simulink model "inverter_hil"  (R2024b)
settings: Solver=FixedStepDiscrete  StartTime=0.0  StopTime=inf  FixedStep=0.001  RelTol=1e-3
InitFcn:
  | enforceHardwarePreflight(bdroot);
values from neighbouring files (symbols this model uses):
  hil_cal_pedals_pressed_v1 = 1.1631952391851683    [inverter_hil.sldd]
  hil_cal_pedals_pressed_v2 = 2.341496910048066    [inverter_hil.sldd]
  hil_cal_pedals_pressed_v3 = 1.6012817578393226    [inverter_hil.sldd]
  hil_cal_pedals_pressed_v4 = 1.6012817578393226    [inverter_hil.sldd]
  hil_cal_pedals_released_v1 = 1.5156786449988555    [inverter_hil.sldd]
  hil_cal_pedals_released_v2 = 3.2025635156786452    [inverter_hil.sldd]
  hil_cal_pedals_released_v3 = 0.45445181963836118    [inverter_hil.sldd]
  hil_cal_pedals_released_v4 = 0.45445181963836118    [inverter_hil.sldd]
  hil_cmd_can_drop_control_mask = 0    [inverter_hil.sldd]
  hil_cmd_can_drop_status_mask = 0    [inverter_hil.sldd]
  hil_cmd_dc_link12_v = 0.0    [inverter_hil.sldd]
  hil_cmd_dc_link34_v = 0.0    [inverter_hil.sldd]
  hil_cmd_digital_cooling_switch = 0    [inverter_hil.sldd]
  hil_cmd_digital_main_button = 0    [inverter_hil.sldd]
  hil_cmd_digital_main_button_sequence = 0    [inverter_hil.sldd]
  hil_cmd_digital_precharge_sequence = 0    [inverter_hil.sldd]
  hil_cmd_digital_shutdown_feedback = 0    [inverter_hil.sldd]
  hil_cmd_gui_heartbeat = 0    [inverter_hil.sldd]
  hil_cmd_imu_dropout = 0    [inverter_hil.sldd]
  hil_cmd_imu_malformed = 0    [inverter_hil.sldd]
  hil_cmd_imu_stale = 0    [inverter_hil.sldd]
  hil_cmd_inverter1_connected = 1    [inverter_hil.sldd]
  hil_cmd_inverter1_fault_mask = 0    [inverter_hil.sldd]
  hil_cmd_inverter1_load_nm = 0.0    [inverter_hil.sldd]
  hil_cmd_inverter2_connected = 1    [inverter_hil.sldd]
  hil_cmd_inverter2_fault_mask = 0    [inverter_hil.sldd]
  hil_cmd_inverter2_load_nm = 0.0    [inverter_hil.sldd]
  hil_cmd_inverter3_connected = 1    [inverter_hil.sldd]
  hil_cmd_inverter3_fault_mask = 0    [inverter_hil.sldd]
  hil_cmd_inverter3_load_nm = 0.0    [inverter_hil.sldd]
  hil_cmd_inverter4_connected = 1    [inverter_hil.sldd]
  hil_cmd_inverter4_fault_mask = 0    [inverter_hil.sldd]
  hil_cmd_inverter4_load_nm = 0.0    [inverter_hil.sldd]
  hil_cmd_pedals_brake = 0.0    [inverter_hil.sldd]
  hil_cmd_pedals_plausibility_override = 0    [inverter_hil.sldd]
  hil_cmd_pedals_throttle = 0.0    [inverter_hil.sldd]
  hil_cmd_steering_angle_deg = 0.0    [inverter_hil.sldd]
  hil_cmd_steering_angle_sentinel = 0    [inverter_hil.sldd]
  hil_cmd_steering_calibration_sequence = 0    [inverter_hil.sldd]
  hil_cmd_steering_dropout = 0    [inverter_hil.sldd]
  hil_cmd_steering_invalid_status = 0    [inverter_hil.sldd]
  hil_cmd_steering_malformed = 0    [inverter_hil.sldd]
  hil_cmd_steering_speed_sentinel = 0    [inverter_hil.sldd]
  hil_cmd_steering_stale = 0    [inverter_hil.sldd]
undefined symbols (not defined in the file or in its folder): Pull, up
libraries: speedgoatlib_IO614 x21, canmsglib x16, speedgoatlib_IO183 x5
(part 2 of 3)

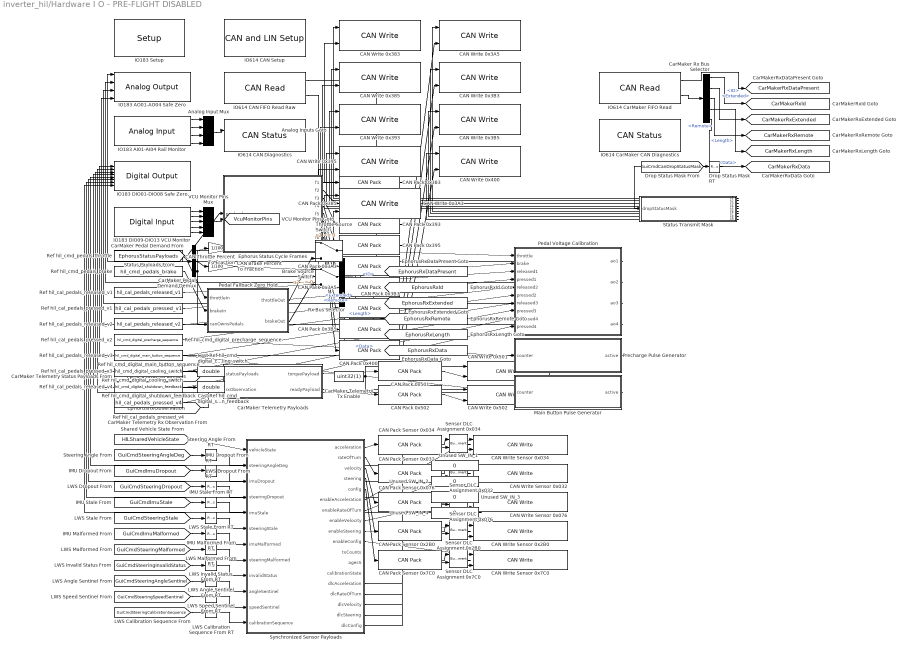
== system inverter_hil/Hardware I O - PRE-FLIGHT DISABLED ==
  Analog Input Mux : Mux
  Brake Source Switch : Switch  Criteria=u2 ~= 0  SaturateOnIntegerOverflow=off  InputSameDT=off
  CAN Brake Percent To Fraction : Gain  Gain=1/100
  CAN Pack 0x383 : canmsglib/CAN Pack  Description=Packs the real status ID 0x383 frame  MsgList=(none)  MsgName=CAN Msg  MsgIDType=Standard (11-bit identifier)  MsgIdentifier=899  CANIDInput=off  MsgLength=8  Remote=off  ApplyMinMax=off  BusOutput=off  SignalInfo={}
      settings: LibrarySourceBlock=canlib/CAN Pack  DataFormat=raw data
  CAN Pack 0x385 : canmsglib/CAN Pack  Description=Packs the real status ID 0x385 frame  MsgList=(none)  MsgName=CAN Msg  MsgIDType=Standard (11-bit identifier)  MsgIdentifier=901  CANIDInput=off  MsgLength=8  Remote=off  ApplyMinMax=off  BusOutput=off  SignalInfo={}
      settings: LibrarySourceBlock=canlib/CAN Pack  DataFormat=raw data
  CAN Pack 0x393 : canmsglib/CAN Pack  Description=Packs the real status ID 0x393 frame  MsgList=(none)  MsgName=CAN Msg  MsgIDType=Standard (11-bit identifier)  MsgIdentifier=915  CANIDInput=off  MsgLength=8  Remote=off  ApplyMinMax=off  BusOutput=off  SignalInfo={}
      settings: LibrarySourceBlock=canlib/CAN Pack  DataFormat=raw data
  CAN Pack 0x395 : canmsglib/CAN Pack  Description=Packs the real status ID 0x395 frame  MsgList=(none)  MsgName=CAN Msg  MsgIDType=Standard (11-bit identifier)  MsgIdentifier=917  CANIDInput=off  MsgLength=8  Remote=off  ApplyMinMax=off  BusOutput=off  SignalInfo={}
      settings: LibrarySourceBlock=canlib/CAN Pack  DataFormat=raw data
  CAN Pack 0x3A3 : canmsglib/CAN Pack  Description=Packs the real status ID 0x3A3 frame  MsgList=(none)  MsgName=CAN Msg  MsgIDType=Standard (11-bit identifier)  MsgIdentifier=931  CANIDInput=off  MsgLength=8  Remote=off  ApplyMinMax=off  BusOutput=off  SignalInfo={}
      settings: LibrarySourceBlock=canlib/CAN Pack  DataFormat=raw data
  CAN Pack 0x3A5 : canmsglib/CAN Pack  Description=Packs the real status ID 0x3A5 frame  MsgList=(none)  MsgName=CAN Msg  MsgIDType=Standard (11-bit identifier)  MsgIdentifier=933  CANIDInput=off  MsgLength=8  Remote=off  ApplyMinMax=off  BusOutput=off  SignalInfo={}
      settings: LibrarySourceBlock=canlib/CAN Pack  DataFormat=raw data
  CAN Pack 0x3B3 : canmsglib/CAN Pack  Description=Packs the real status ID 0x3B3 frame  MsgList=(none)  MsgName=CAN Msg  MsgIDType=Standard (11-bit identifier)  MsgIdentifier=947  CANIDInput=off  MsgLength=8  Remote=off  ApplyMinMax=off  BusOutput=off  SignalInfo={}
      settings: LibrarySourceBlock=canlib/CAN Pack  DataFormat=raw data
  CAN Pack 0x3B5 : canmsglib/CAN Pack  Description=Packs the real status ID 0x3B5 frame  MsgList=(none)  MsgName=CAN Msg  MsgIDType=Standard (11-bit identifier)  MsgIdentifier=949  CANIDInput=off  MsgLength=8  Remote=off  ApplyMinMax=off  BusOutput=off  SignalInfo={}
      settings: LibrarySourceBlock=canlib/CAN Pack  DataFormat=raw data
  CAN Pack 0x400 : canmsglib/CAN Pack  Description=Packs the real status ID 0x400 frame  MsgList=(none)  MsgName=CAN Msg  MsgIDType=Standard (11-bit identifier)  MsgIdentifier=1024  CANIDInput=off  MsgLength=8  Remote=off  ApplyMinMax=off  BusOutput=off  SignalInfo={}
      settings: LibrarySourceBlock=canlib/CAN Pack  DataFormat=raw data
  CAN Pack 0x501 : canmsglib/CAN Pack  Description=Packs CarMaker telemetry ID 0x501  MsgList=(none)  MsgName=CAN Msg  MsgIDType=Standard (11-bit identifier)  MsgIdentifier=1281  CANIDInput=off  MsgLength=8  Remote=off  ApplyMinMax=off  BusOutput=off  SignalInfo={}
      settings: LibrarySourceBlock=canlib/CAN Pack  DataFormat=raw data
  CAN Pack 0x502 : canmsglib/CAN Pack  Description=Packs CarMaker telemetry ID 0x502  MsgList=(none)  MsgName=CAN Msg  MsgIDType=Standard (11-bit identifier)  MsgIdentifier=1282  CANIDInput=off  MsgLength=8  Remote=off  ApplyMinMax=off  BusOutput=off  SignalInfo={}
      settings: LibrarySourceBlock=canlib/CAN Pack  DataFormat=raw data
  CAN Pack Sensor 0x032 : canmsglib/CAN Pack  Description=Packs independent sensor ID 0x032  MsgList=(none)  MsgName=CAN Msg  MsgIDType=Standard (11-bit identifier)  MsgIdentifier=50  CANIDInput=off  MsgLength=6  Remote=off  ApplyMinMax=off  BusOutput=on  SignalInfo={}
      settings: LibrarySourceBlock=canlib/CAN Pack  DataFormat=raw data
  CAN Pack Sensor 0x034 : canmsglib/CAN Pack  Description=Packs independent sensor ID 0x034  MsgList=(none)  MsgName=CAN Msg  MsgIDType=Standard (11-bit identifier)  MsgIdentifier=52  CANIDInput=off  MsgLength=6  Remote=off  ApplyMinMax=off  BusOutput=on  SignalInfo={}
      settings: LibrarySourceBlock=canlib/CAN Pack  DataFormat=raw data
  CAN Pack Sensor 0x076 : canmsglib/CAN Pack  Description=Packs independent sensor ID 0x076  MsgList=(none)  MsgName=CAN Msg  MsgIDType=Standard (11-bit identifier)  MsgIdentifier=118  CANIDInput=off  MsgLength=6  Remote=off  ApplyMinMax=off  BusOutput=on  SignalInfo={}
      settings: LibrarySourceBlock=canlib/CAN Pack  DataFormat=raw data
  CAN Pack Sensor 0x2B0 : canmsglib/CAN Pack  Description=Packs independent sensor ID 0x2B0  MsgList=(none)  MsgName=CAN Msg  MsgIDType=Standard (11-bit identifier)  MsgIdentifier=688  CANIDInput=off  MsgLength=5  Remote=off  ApplyMinMax=off  BusOutput=on  SignalInfo={}
      settings: LibrarySourceBlock=canlib/CAN Pack  DataFormat=raw data
  CAN Pack Sensor 0x7C0 : canmsglib/CAN Pack  Description=Packs independent sensor ID 0x7C0  MsgList=(none)  MsgName=CAN Msg  MsgIDType=Standard (11-bit identifier)  MsgIdentifier=1984  CANIDInput=off  MsgLength=2  Remote=off  ApplyMinMax=off  BusOutput=on  SignalInfo={}
      settings: LibrarySourceBlock=canlib/CAN Pack  DataFormat=raw data
  CAN Throttle Percent To Fraction : Gain  Gain=1/100
  CAN Write 0x383 : speedgoatlib_IO614/CAN Write   Description=Ordered Ephorus status ID 0x383  moduleType=IO614  id=1  channel=2  canType=CAN (HS)  useBusIn=off  numOfMsg=1  enableInput=on  enableStatusPort=on  initValues=[614 1 0.005 1 1 1 1 1 1 0]  ts=0.005
  CAN Write 0x385 : speedgoatlib_IO614/CAN Write   Description=Ordered Ephorus status ID 0x385  moduleType=IO614  id=1  channel=2  canType=CAN (HS)  useBusIn=off  numOfMsg=1  enableInput=on  enableStatusPort=on  initValues=[614 1 0.005 1 1 1 1 1 1 0]  ts=0.005
  CAN Write 0x393 : speedgoatlib_IO614/CAN Write   Description=Ordered Ephorus status ID 0x393  moduleType=IO614  id=1  channel=2  canType=CAN (HS)  useBusIn=off  numOfMsg=1  enableInput=on  enableStatusPort=on  initValues=[614 1 0.005 1 1 1 1 1 1 0]  ts=0.005
  CAN Write 0x395 : speedgoatlib_IO614/CAN Write   Description=Ordered Ephorus status ID 0x395  moduleType=IO614  id=1  channel=2  canType=CAN (HS)  useBusIn=off  numOfMsg=1  enableInput=on  enableStatusPort=on  initValues=[614 1 0.005 1 1 1 1 1 1 0]  ts=0.005
  CAN Write 0x3A3 : speedgoatlib_IO614/CAN Write   Description=Ordered Ephorus status ID 0x3A3  moduleType=IO614  id=1  channel=2  canType=CAN (HS)  useBusIn=off  numOfMsg=1  enableInput=on  enableStatusPort=on  initValues=[614 1 0.005 1 1 1 1 1 1 0]  ts=0.005
  CAN Write 0x3A5 : speedgoatlib_IO614/CAN Write   Description=Ordered Ephorus status ID 0x3A5  moduleType=IO614  id=1  channel=2  canType=CAN (HS)  useBusIn=off  numOfMsg=1  enableInput=on  enableStatusPort=on  initValues=[614 1 0.005 1 1 1 1 1 1 0]  ts=0.005
  CAN Write 0x3B3 : speedgoatlib_IO614/CAN Write   Description=Ordered Ephorus status ID 0x3B3  moduleType=IO614  id=1  channel=2  canType=CAN (HS)  useBusIn=off  numOfMsg=1  enableInput=on  enableStatusPort=on  initValues=[614 1 0.005 1 1 1 1 1 1 0]  ts=0.005
  CAN Write 0x3B5 : speedgoatlib_IO614/CAN Write   Description=Ordered Ephorus status ID 0x3B5  moduleType=IO614  id=1  channel=2  canType=CAN (HS)  useBusIn=off  numOfMsg=1  enableInput=on  enableStatusPort=on  initValues=[614 1 0.005 1 1 1 1 1 1 0]  ts=0.005
  CAN Write 0x400 : speedgoatlib_IO614/CAN Write   Description=Ordered Ephorus status ID 0x400  moduleType=IO614  id=1  channel=2  canType=CAN (HS)  useBusIn=off  numOfMsg=1  enableInput=on  enableStatusPort=on  initValues=[614 1 0.005 1 1 1 1 1 1 0]  ts=0.005
  CAN Write 0x501 : speedgoatlib_IO614/CAN Write   Description=Transmits CarMaker telemetry ID 0x501  moduleType=IO614  id=1  channel=1  canType=CAN (HS)  useBusIn=off  numOfMsg=1  enableInput=on  enableStatusPort=on  initValues=[614 1 0.005 0 1 1 1 1 1 0]  ts=0.005
  CAN Write 0x502 : speedgoatlib_IO614/CAN Write   Description=Transmits CarMaker telemetry ID 0x502  moduleType=IO614  id=1  channel=1  canType=CAN (HS)  useBusIn=off  numOfMsg=1  enableInput=on  enableStatusPort=on  initValues=[614 1 0.005 0 1 1 1 1 1 0]  ts=0.005
  CAN Write Sensor 0x032 : speedgoatlib_IO614/CAN Write   Description=Transmits independent sensor ID 0x032  moduleType=IO614  id=1  channel=2  canType=CAN (HS)  useBusIn=on  numOfMsg=1  enableInput=on  enableStatusPort=on  initValues=[614 1 0.005 1 1 1 1 1 1 1]  ts=0.005
  CAN Write Sensor 0x034 : speedgoatlib_IO614/CAN Write   Description=Transmits independent sensor ID 0x034  moduleType=IO614  id=1  channel=2  canType=CAN (HS)  useBusIn=on  numOfMsg=1  enableInput=on  enableStatusPort=on  initValues=[614 1 0.005 1 1 1 1 1 1 1]  ts=0.005
  CAN Write Sensor 0x076 : speedgoatlib_IO614/CAN Write   Description=Transmits independent sensor ID 0x076  moduleType=IO614  id=1  channel=2  canType=CAN (HS)  useBusIn=on  numOfMsg=1  enableInput=on  enableStatusPort=on  initValues=[614 1 0.005 1 1 1 1 1 1 1]  ts=0.005
  CAN Write Sensor 0x2B0 : speedgoatlib_IO614/CAN Write   Description=Transmits independent sensor ID 0x2B0  moduleType=IO614  id=1  channel=2  canType=CAN (HS)  useBusIn=on  numOfMsg=1  enableInput=on  enableStatusPort=on  initValues=[614 1 0.005 1 1 1 1 1 1 1]  ts=0.005
  CAN Write Sensor 0x7C0 : speedgoatlib_IO614/CAN Write   Description=Transmits independent sensor ID 0x7C0  moduleType=IO614  id=1  channel=2  canType=CAN (HS)  useBusIn=on  numOfMsg=1  enableInput=on  enableStatusPort=on  initValues=[614 1 0.005 1 1 1 1 1 1 1]  ts=0.005
  CarMaker Pedal Demand Demux : Demux  Outputs=3
  CarMaker Rx Bus Selector : BusSelector  OutputSignals=ID,Extended,Remote,Length,Data
  CarMaker Telemetry Payloads : MATLAB Function  TreatAsAtomicUnit=on
  CarMaker Telemetry Tx Enable : Constant  Value=uint32(1)  SampleTime=0.005
  Cast Ref hil_cmd_digital_cooling_switch : DataTypeConversion  OutDataTypeStr=double  SaturateOnIntegerOverflow=off  RndMeth=Floor
  Cast Ref hil_cmd_digital_shutdown_feedback : DataTypeConversion  OutDataTypeStr=double  SaturateOnIntegerOverflow=off  RndMeth=Floor
  Drop Status Mask RT : RateTransition
  Ephorus Status Cycle Frames : MATLAB Function  TreatAsAtomicUnit=on
  IMU Dropout From RT : RateTransition
  IMU Malformed From RT : RateTransition
  IMU Stale From RT : RateTransition
  IO183 AI01-AI04 Rail Monitor : speedgoatlib_IO183/Analog Input  Priority=0  parModuleId=1  parSampTime=0.001  parPciSlot=-1  parAdChannelLow=1  parAdChannelHigh=4
  IO183 AO01-AO04 Safe Zero : speedgoatlib_IO183/Analog Output  parModuleId=1  parSampTime=0.001  parDaSimult=on  parPciSlot=-1  parDaChannels=[1 2 3 4]  parDaInit=[0 0 0 0]  parDaReset=[0 0 0 0]
  IO183 DIO01-DIO08 Safe Zero : speedgoatlib_IO183/Digital Output  parModuleId=1  parSampTime=0.001  parPciSlot=-1  parDoChannels=[1 2 3 4 5 6 7 8]  parDoInit=[0 0 0 0 0 0 0 0]  parDoReset=[0 0 0 0 0 0 0 0]
  IO183 DIO09-DIO13 VCU Monitor : speedgoatlib_IO183/Digital Input  parModuleId=1  parSampTime=0.001  parPciSlot=-1  parDiChannels=[9 10 11 12 13]
  IO183 Setup : speedgoatlib_IO183/Setup  parModuleId=1  parPciSlot=-1  parDaSimult=on  parAdCoupling=Single Ended  parAdRange=0..5V  parAdChannelLow=1  parAdChannelHigh=4  parDaChannels=[1 2 3 4]  parDaRange=0..5V  parDaInit=[0 0 0 0]  parDaReset=[0 0 0 0]  parDoChannels=[1 2 3 4 5 6 7 8]  parDoInit=[0 0 0 0 0 0 0 0]  parDoReset=[0 0 0 0 0 0 0 0]  parDiChannels=[9 10 11 12 13]  parIOPullReferenceFront=Pull-down  parIOPullReferenceRear=Pull-up (3.3V)
  IO614 CAN Diagnostics : speedgoatlib_IO614/CAN Status   moduleType=IO614  id=1  channel=2  canType=CAN (HS)  autoRecovery=off  enableInput=off  ts=0.001  initValues=[614 1 0.001 1 0 0 0 0 0 0 0 0 0 0 0]
      settings: LibrarySourceBlock=speedgoatlib_CANLIN_OfA2/CAN/CAN Status
  IO614 CAN FIFO Read Raw : speedgoatlib_IO614/CAN Read   moduleType=IO614  id=1  channel=2  canType=CAN (HS)  useBusOut=on  HasMulRead=Single Read from Buffer (FIFO)  MsgIDlist=[1 2]  isEFF=off  LabelInHex=on  enableInput=off  ts=0.001  initValues=[614 1 0.001 1 1 1 0 1 0 1 2 1 2]
  IO614 CAN Setup : speedgoatlib_IO614/CAN and LIN Setup   moduleInitValues="[614    1    1   -1   -1]"  id=1  moduleType=IO614  pciSlot=-1  canChn1=CAN (HS)  canChn2=CAN (HS)  canChn3=Disabled  canChn4=Disabled  linChn1=Disabled  linChn2=Disabled  canInitStructArray=[]  canTermStructArray=[]  canChn1InitValues="[2   2   1  31   8   2   1   5   2]"  arbBdrChn1=1.0 MBaud  arbManBdrChn1=[2,1,31,8]  fdBdrChn1=5.0 MBaud  fdManBdrChn1=[2,1,5,2]  canChn2InitValues="[2   2   1  31   8   2   1   5   2]"  arbBdrChn2=1.0 MBaud  arbManBdrChn2=[2,1,31,8]  fdBdrChn2=5.0 MBaud  fdManBdrChn2=[2,1,5,2]  canChn3InitValues="[1   2   1  31   8   2   1   5   2]"  arbBdrChn3=1.0 MBaud  arbManBdrChn3=[2,1,31,8]  fdBdrChn3=5.0 MBaud  fdManBdrChn3=[2,1,5,2]  canChn4InitValues="[1   2   1  31   8   2   1   5   2]"  arbBdrChn4=1.0 MBaud  arbManBdrChn4=[2,1,31,8]  fdBdrChn4=5.0 MBaud  fdManBdrChn4=[2,1,5,2]  bdrLIN1=19200  linChn1InitValues="[1  19200]"  bdrLIN2=19200  linChn2InitValues="[1  19200]"
      settings: LibrarySourceBlock=speedgoatlib_CANLIN_OfA2/CAN and LIN Setup
  IO614 CarMaker CAN Diagnostics : speedgoatlib_IO614/CAN Status   moduleType=IO614  id=1  channel=1  canType=CAN (HS)  autoRecovery=off  enableInput=off  ts=0.001  initValues=[614 1 0.001 0 0 0 0 0 0 0 0 0 0 0 0]
      settings: LibrarySourceBlock=speedgoatlib_CANLIN_OfA2/CAN/CAN Status
  IO614 CarMaker FIFO Read : speedgoatlib_IO614/CAN Read   moduleType=IO614  id=1  channel=1  canType=CAN (HS)  useBusOut=on  HasMulRead=Single Read from Buffer (FIFO)  MsgIDlist=[1 2]  isEFF=off  LabelInHex=on  enableInput=off  ts=0.001  initValues=[614 1 0.001 0 1 1 0 1 0 1 2 1 2]
  LWS Angle Sentinel From RT : RateTransition
  LWS Calibration Sequence From RT : RateTransition
  LWS Dropout From RT : RateTransition
  LWS Invalid Status From RT : RateTransition
  LWS Malformed From RT : RateTransition
  LWS Speed Sentinel From RT : RateTransition
  LWS Stale From RT : RateTransition
  Main Button Pulse Generator : MATLAB Function  TreatAsAtomicUnit=on
  Pedal Fallback Zero Hold : MATLAB Function  TreatAsAtomicUnit=on
  Pedal Voltage Calibration : MATLAB Function  TreatAsAtomicUnit=on
  Precharge Pulse Generator : MATLAB Function  TreatAsAtomicUnit=on
  Ref hil_cal_pedals_pressed_v1 : Constant  Value=hil_cal_pedals_pressed_v1  SampleTime=0.001
  Ref hil_cal_pedals_pressed_v2 : Constant  Value=hil_cal_pedals_pressed_v2  SampleTime=0.001
  Ref hil_cal_pedals_pressed_v3 : Constant  Value=hil_cal_pedals_pressed_v3  SampleTime=0.001
  Ref hil_cal_pedals_pressed_v4 : Constant  Value=hil_cal_pedals_pressed_v4  SampleTime=0.001
  Ref hil_cal_pedals_released_v1 : Constant  Value=hil_cal_pedals_released_v1  SampleTime=0.001
  Ref hil_cal_pedals_released_v2 : Constant  Value=hil_cal_pedals_released_v2  SampleTime=0.001
  Ref hil_cal_pedals_released_v3 : Constant  Value=hil_cal_pedals_released_v3  SampleTime=0.001
  Ref hil_cal_pedals_released_v4 : Constant  Value=hil_cal_pedals_released_v4  SampleTime=0.001
  Ref hil_cmd_digital_cooling_switch : Constant  Value=hil_cmd_digital_cooling_switch  OutDataTypeStr=boolean  SampleTime=0.001
  Ref hil_cmd_digital_main_button_sequence : Constant  Value=hil_cmd_digital_main_button_sequence  OutDataTypeStr=uint32  SampleTime=0.001
  Ref hil_cmd_digital_precharge_sequence : Constant  Value=hil_cmd_digital_precharge_sequence  OutDataTypeStr=uint32  SampleTime=0.001
  Ref hil_cmd_digital_shutdown_feedback : Constant  Value=hil_cmd_digital_shutdown_feedback  OutDataTypeStr=boolean  SampleTime=0.001
  Ref hil_cmd_pedals_brake : Constant  Value=hil_cmd_pedals_brake  SampleTime=0.001
  Ref hil_cmd_pedals_throttle : Constant  Value=hil_cmd_pedals_throttle  SampleTime=0.001
  Rx Bus Selector : BusSelector  OutputSignals=ID,Extended,Remote,Length,Data
  Sensor DLC Assignment 0x032 : BusAssignment  AssignedSignals=Length
  Sensor DLC Assignment 0x034 : BusAssignment  AssignedSignals=Length
  Sensor DLC Assignment 0x076 : BusAssignment  AssignedSignals=Length
  Sensor DLC Assignment 0x2B0 : BusAssignment  AssignedSignals=Length
  Sensor DLC Assignment 0x7C0 : BusAssignment  AssignedSignals=Length
  Status Transmit Mask : MATLAB Function  TreatAsAtomicUnit=on
  Steering Angle From RT : RateTransition
  Synchronized Sensor Payloads : MATLAB Function  TreatAsAtomicUnit=on
  Throttle Source Switch : Switch  Criteria=u2 ~= 0  SaturateOnIntegerOverflow=off  InputSameDT=off
  Unused SW_IN_{1..4} (4 alike) : Constant  Value=0  OutDataTypeStr=double  SampleTime=0.001
  VCU Monitor Pins Mux : Mux  Inputs=5
  tag scope: AnalogInputsV=global, CarMakerRxData=global, CarMakerRxDataPresent=global, CarMakerRxExtended=global, CarMakerRxId=global, CarMakerRxLength=global, CarMakerRxRemote=global, EphorusRxData=global, EphorusRxDataPresent=global, EphorusRxExtended=global, EphorusRxId=global, EphorusRxLength=global, EphorusRxRemote=global, VcuMonitorPins=global
  wires:
  ? -> ?
  IO183 AI01-AI04 Rail Monitor/1 -> Analog Input Mux/1
  IO183 AI01-AI04 Rail Monitor/2 -> Analog Input Mux/2
  IO183 AI01-AI04 Rail Monitor/3 -> Analog Input Mux/3
  IO183 AI01-AI04 Rail Monitor/4 -> Analog Input Mux/4
  Analog Input Mux/1 -> [AnalogInputsV]
  IO183 DIO09-DIO13 VCU Monitor/1 -> VCU Monitor Pins Mux/1
  IO183 DIO09-DIO13 VCU Monitor/2 -> VCU Monitor Pins Mux/2
  IO183 DIO09-DIO13 VCU Monitor/3 -> VCU Monitor Pins Mux/3
  IO183 DIO09-DIO13 VCU Monitor/4 -> VCU Monitor Pins Mux/4
  IO183 DIO09-DIO13 VCU Monitor/5 -> VCU Monitor Pins Mux/5
  VCU Monitor Pins Mux/1 -> [VcuMonitorPins]
  IO614 CAN FIFO Read Raw/2 -> Rx Bus Selector/1
  IO614 CAN FIFO Read Raw/1 -> [EphorusRxDataPresent]
  Rx Bus Selector/1 -> [EphorusRxId]  "<ID>"
  Rx Bus Selector/2 -> [EphorusRxExtended]  "<Extended>"
  Rx Bus Selector/3 -> [EphorusRxRemote]  "<Remote>"
  Rx Bus Selector/4 -> [EphorusRxLength]  "<Length>"
  Rx Bus Selector/5 -> [EphorusRxData]  "<Data>"
  IO614 CarMaker FIFO Read/2 -> CarMaker Rx Bus Selector/1
  IO614 CarMaker FIFO Read/1 -> [CarMakerRxDataPresent]
  CarMaker Rx Bus Selector/1 -> [CarMakerRxId]  "<ID>"
  CarMaker Rx Bus Selector/2 -> [CarMakerRxExtended]  "<Extended>"
  CarMaker Rx Bus Selector/3 -> [CarMakerRxRemote]  "<Remote>"
  CarMaker Rx Bus Selector/4 -> [CarMakerRxLength]  "<Length>"
  CarMaker Rx Bus Selector/5 -> [CarMakerRxData]  "<Data>"
  [HILSharedVehicleState] -> Synchronized Sensor Payloads/1(vehicleState)
  [GuiCmdSteeringAngleDeg] -> Steering Angle From RT/1
  Steering Angle From RT/1 -> Synchronized Sensor Payloads/2(steeringAngleDeg)
  [GuiCmdImuDropout] -> IMU Dropout From RT/1
  IMU Dropout From RT/1 -> Synchronized Sensor Payloads/3(imuDropout)
  [GuiCmdSteeringDropout] -> LWS Dropout From RT/1
  LWS Dropout From RT/1 -> Synchronized Sensor Payloads/4(steeringDropout)
  [GuiCmdImuStale] -> IMU Stale From RT/1
  IMU Stale From RT/1 -> Synchronized Sensor Payloads/5(imuStale)
  [GuiCmdSteeringStale] -> LWS Stale From RT/1
  LWS Stale From RT/1 -> Synchronized Sensor Payloads/6(steeringStale)
  [GuiCmdImuMalformed] -> IMU Malformed From RT/1
  IMU Malformed From RT/1 -> Synchronized Sensor Payloads/7(imuMalformed)
  [GuiCmdSteeringMalformed] -> LWS Malformed From RT/1
  LWS Malformed From RT/1 -> Synchronized Sensor Payloads/8(steeringMalformed)
  [GuiCmdSteeringInvalidStatus] -> LWS Invalid Status From RT/1
  LWS Invalid Status From RT/1 -> Synchronized Sensor Payloads/9(invalidStatus)
  [GuiCmdSteeringAngleSentinel] -> LWS Angle Sentinel From RT/1
  LWS Angle Sentinel From RT/1 -> Synchronized Sensor Payloads/10(angleSentinel)
  [GuiCmdSteeringSpeedSentinel] -> LWS Speed Sentinel From RT/1
  LWS Speed Sentinel From RT/1 -> Synchronized Sensor Payloads/11(speedSentinel)
  [GuiCmdSteeringCalibrationSequence] -> LWS Calibration Sequence From RT/1
  LWS Calibration Sequence From RT/1 -> Synchronized Sensor Payloads/12(calibrationSequence)
  Synchronized Sensor Payloads/1(acceleration) -> CAN Pack Sensor 0x034/1
  CAN Pack Sensor 0x034/1 -> Sensor DLC Assignment 0x034/1
  Synchronized Sensor Payloads/14(dlcAcceleration) -> Sensor DLC Assignment 0x034/2
  Synchronized Sensor Payloads/6(enableAcceleration) -> CAN Write Sensor 0x034/1
  Sensor DLC Assignment 0x034/1 -> CAN Write Sensor 0x034/2
  Synchronized Sensor Payloads/2(rateOfTurn) -> CAN Pack Sensor 0x032/1
  CAN Pack Sensor 0x032/1 -> Sensor DLC Assignment 0x032/1
  Synchronized Sensor Payloads/15(dlcRateOfTurn) -> Sensor DLC Assignment 0x032/2
  Synchronized Sensor Payloads/7(enableRateOfTurn) -> CAN Write Sensor 0x032/1
  Sensor DLC Assignment 0x032/1 -> CAN Write Sensor 0x032/2
  Synchronized Sensor Payloads/3(velocity) -> CAN Pack Sensor 0x076/1
  CAN Pack Sensor 0x076/1 -> Sensor DLC Assignment 0x076/1
  Synchronized Sensor Payloads/16(dlcVelocity) -> Sensor DLC Assignment 0x076/2
  Synchronized Sensor Payloads/8(enableVelocity) -> CAN Write Sensor 0x076/1
  Sensor DLC Assignment 0x076/1 -> CAN Write Sensor 0x076/2
  Synchronized Sensor Payloads/4(steering) -> CAN Pack Sensor 0x2B0/1
  CAN Pack Sensor 0x2B0/1 -> Sensor DLC Assignment 0x2B0/1
  Synchronized Sensor Payloads/17(dlcSteering) -> Sensor DLC Assignment 0x2B0/2
  Synchronized Sensor Payloads/9(enableSteering) -> CAN Write Sensor 0x2B0/1
  Sensor DLC Assignment 0x2B0/1 -> CAN Write Sensor 0x2B0/2
  Synchronized Sensor Payloads/5(config) -> CAN Pack Sensor 0x7C0/1
  CAN Pack Sensor 0x7C0/1 -> Sensor DLC Assignment 0x7C0/1
  Synchronized Sensor Payloads/18(dlcConfig) -> Sensor DLC Assignment 0x7C0/2
  Synchronized Sensor Payloads/10(enableConfig) -> CAN Write Sensor 0x7C0/1
  Sensor DLC Assignment 0x7C0/1 -> CAN Write Sensor 0x7C0/2
  [GuiCmdCanDropStatusMask] -> Drop Status Mask RT/1
  Drop Status Mask RT/1 -> Status Transmit Mask/1(dropStatusMask)
  Status Transmit Mask/1(k1) -> CAN Write 0x383/1
  Status Transmit Mask/2(k2) -> CAN Write 0x385/1
  Status Transmit Mask/3(k3) -> CAN Write 0x393/1
  Status Transmit Mask/4(k4) -> CAN Write 0x395/1
  Status Transmit Mask/5(k5) -> CAN Write 0x3A3/1
  Status Transmit Mask/6(k6) -> CAN Write 0x3A5/1
  Status Transmit Mask/7(k7) -> CAN Write 0x3B3/1
  Status Transmit Mask/8(k8) -> CAN Write 0x3B5/1
  Status Transmit Mask/9(k9) -> CAN Write 0x400/1
  [EphorusStatusPayloads] -> Ephorus Status Cycle Frames/1(payloads)
  Ephorus Status Cycle Frames/1(f1) -> CAN Pack 0x383/1
  CAN Pack 0x383/1 -> CAN Write 0x383/2
  Ephorus Status Cycle Frames/2(f2) -> CAN Pack 0x385/1
  CAN Pack 0x385/1 -> CAN Write 0x385/2
  Ephorus Status Cycle Frames/3(f3) -> CAN Pack 0x393/1
  CAN Pack 0x393/1 -> CAN Write 0x393/2
  Ephorus Status Cycle Frames/4(f4) -> CAN Pack 0x395/1
  CAN Pack 0x395/1 -> CAN Write 0x395/2
  Ephorus Status Cycle Frames/5(f5) -> CAN Pack 0x3A3/1
  CAN Pack 0x3A3/1 -> CAN Write 0x3A3/2
  Ephorus Status Cycle Frames/6(f6) -> CAN Pack 0x3A5/1
  CAN Pack 0x3A5/1 -> CAN Write 0x3A5/2
  Ephorus Status Cycle Frames/7(f7) -> CAN Pack 0x3B3/1
  CAN Pack 0x3B3/1 -> CAN Write 0x3B3/2
  Ephorus Status Cycle Frames/8(f8) -> CAN Pack 0x3B5/1
  CAN Pack 0x3B5/1 -> CAN Write 0x3B5/2
  Ephorus Status Cycle Frames/9(f9) -> CAN Pack 0x400/1
  CAN Pack 0x400/1 -> CAN Write 0x400/2
  [EphorusStatusPayloads] -> CarMaker Telemetry Payloads/1(statusPayloads)
  [EphorusRxObservation] -> CarMaker Telemetry Payloads/2(rxObservation)
  CarMaker Telemetry Payloads/1(torquePayload) -> CAN Pack 0x501/1
  CarMaker Telemetry Tx Enable/1 -> CAN Write 0x501/1, CAN Write 0x502/1
  CAN Pack 0x501/1 -> CAN Write 0x501/2
  CarMaker Telemetry Payloads/2(readyPayload) -> CAN Pack 0x502/1
  CAN Pack 0x502/1 -> CAN Write 0x502/2
  [CarMakerPedalDemand] -> CarMaker Pedal Demand Demux/1
  CarMaker Pedal Demand Demux/1 -> CAN Throttle Percent To Fraction/1
  CarMaker Pedal Demand Demux/2 -> CAN Brake Percent To Fraction/1
  Ref hil_cmd_pedals_throttle/1 -> Pedal Fallback Zero Hold/1(throttleIn)
  Ref hil_cmd_pedals_brake/1 -> Pedal Fallback Zero Hold/2(brakeIn)
  CarMaker Pedal Demand Demux/3 -> Pedal Fallback Zero Hold/3(canOwnsPedals), Throttle Source Switch/2, Brake Source Switch/2
  CAN Throttle Percent To Fraction/1 -> Throttle Source Switch/1
  Pedal Fallback Zero Hold/1(throttleOut) -> Throttle Source Switch/3
  CAN Brake Percent To Fraction/1 -> Brake Source Switch/1
  Pedal Fallback Zero Hold/2(brakeOut) -> Brake Source Switch/3
  Throttle Source Switch/1 -> Pedal Voltage Calibration/1(throttle)
  Brake Source Switch/1 -> Pedal Voltage Calibration/2(brake)
  Ref hil_cal_pedals_released_v1/1 -> Pedal Voltage Calibration/3(released1)
  Ref hil_cal_pedals_pressed_v1/1 -> Pedal Voltage Calibration/4(pressed1)
  Ref hil_cal_pedals_released_v2/1 -> Pedal Voltage Calibration/5(released2)
  Ref hil_cal_pedals_pressed_v2/1 -> Pedal Voltage Calibration/6(pressed2)
  Ref hil_cal_pedals_released_v3/1 -> Pedal Voltage Calibration/7(released3)
  Ref hil_cal_pedals_pressed_v3/1 -> Pedal Voltage Calibration/8(pressed3)
  Ref hil_cal_pedals_released_v4/1 -> Pedal Voltage Calibration/9(released4)
  Ref hil_cal_pedals_pressed_v4/1 -> Pedal Voltage Calibration/10(pressed4)
  Pedal Voltage Calibration/1(ao1) -> IO183 AO01-AO04 Safe Zero/1
  Pedal Voltage Calibration/2(ao2) -> IO183 AO01-AO04 Safe Zero/2
  Pedal Voltage Calibration/3(ao3) -> IO183 AO01-AO04 Safe Zero/3
  Pedal Voltage Calibration/4(ao4) -> IO183 AO01-AO04 Safe Zero/4
  Ref hil_cmd_digital_precharge_sequence/1 -> Precharge Pulse Generator/1(counter)
  Precharge Pulse Generator/1(active) -> IO183 DIO01-DIO08 Safe Zero/1
  Ref hil_cmd_digital_main_button_sequence/1 -> Main Button Pulse Generator/1(counter)
  Main Button Pulse Generator/1(active) -> IO183 DIO01-DIO08 Safe Zero/2
  Ref hil_cmd_digital_cooling_switch/1 -> Cast Ref hil_cmd_digital_cooling_switch/1
  Cast Ref hil_cmd_digital_cooling_switch/1 -> IO183 DIO01-DIO08 Safe Zero/3
  Ref hil_cmd_digital_shutdown_feedback/1 -> Cast Ref hil_cmd_digital_shutdown_feedback/1
  Cast Ref hil_cmd_digital_shutdown_feedback/1 -> IO183 DIO01-DIO08 Safe Zero/4
  Unused SW_IN_1/1 -> IO183 DIO01-DIO08 Safe Zero/5
  Unused SW_IN_2/1 -> IO183 DIO01-DIO08 Safe Zero/6
  Unused SW_IN_3/1 -> IO183 DIO01-DIO08 Safe Zero/7
  Unused SW_IN_4/1 -> IO183 DIO01-DIO08 Safe Zero/8

== matlab function inverter_hil/Hardware I O - PRE-FLIGHT DISABLED/Status Transmit Mask ==
  data: dropStatusMask input; k1 output; k2 output; k3 output; k4 output; k5 output; k6 output; k7 output; k8 output; k9 output
function [k1,k2,k3,k4,k5,k6,k7,k8,k9] = ...
    ephorusStatusTransmitMask(dropStatusMask)
%#codegen
%EPHORUSSTATUSTRANSMITMASK Fix 4: split INVERTERHIL.STATUSTRANSMITMASK's
%9-entry keep vector into nine scalar Tx Control outputs, one per
%CAN Write block in INVERTERHIL.PROTOCOL status-cycle order, because
%each CAN Write's Tx Control port takes a scalar and a MATLAB
%Function block cannot emit a bus without a Simulink.Bus definition.
%
%CAN Write's Tx Control input is uint32 (a transmit-count control, not
%a boolean enable), so KEEP is cast rather than passed as logical: 1 to
%transmit this tick, 0 to genuinely skip it.
keep = uint32(statusTransmitMask(dropStatusMask));
k1 = keep(1); k2 = keep(2); k3 = keep(3);
k4 = keep(4); k5 = keep(5); k6 = keep(6);
k7 = keep(7); k8 = keep(8); k9 = keep(9);
end

== matlab function inverter_hil/Hardware I O - PRE-FLIGHT DISABLED/Ephorus Status Cycle Frames ==
  data: payloads input; f1 output; f2 output; f3 output; f4 output; f5 output; f6 output; f7 output; f8 output; f9 output
function [f1,f2,f3,f4,f5,f6,f7,f8,f9] = ephorusStatusCycleFrames(payloads)
%EPHORUSSTATUSCYCLEFRAMES Split the nine-frame status cycle into the
%nine 1x8 rows the CAN Pack blocks need, one per status ID, in the
%order INVERTERHIL.PROTOCOL declares.
f1 = payloads(1,:); f2 = payloads(2,:); f3 = payloads(3,:);
f4 = payloads(4,:); f5 = payloads(5,:); f6 = payloads(6,:);
f7 = payloads(7,:); f8 = payloads(8,:); f9 = payloads(9,:);
end

== matlab function inverter_hil/Hardware I O - PRE-FLIGHT DISABLED/CarMaker Telemetry Payloads ==
  data: statusPayloads input; torquePayload output; rxObservation input; readyPayload output
function [torquePayload, readyPayload] = carMakerTelemetryPayloads( ...
    statusPayloads, rxObservation)
%#codegen
%CARMAKERTELEMETRYPAYLOADS Derive the compact CarMaker contract.
%TORQUESETPOINTNM is the VC's own commanded torque limit, decoded
%straight from RXOBSERVATION's retained control-frame rows (1:4,
%columns 1:8) with the SAME INVERTERHIL.DECODECONTROLFRAME
%EPHORUSSYSTEMSTATUSSTEP itself uses -- not re-derived from
%Speedgoat's own simulated 3X3 status echo, which reports what a
%simulated inverter would answer, not what the VC asked for.
%READY is unchanged: still the 3X3 status payloads' own
%InverterReady bit.
torqueSetpointNm = zeros(1, 4);
ready = false(1, 4);
controlIds = protocol().controlIds;
for channel = 1:4
    status = decodeStatus3X3(statusPayloads(2 * channel - 1, :));
    ready(channel) = status.ready;
    hasCommand = rxObservation(channel, 9) ~= 0;
    if hasCommand
        framePayload = uint8(rxObservation(channel, 1:8));
        [~, ~, command] = decodeControlFrame( ...
            controlIds(channel), uint8(8), framePayload, false, false);
        torqueSetpointNm(channel) = command.torquePosNm256;
    end
end
telemetry.torqueSetpointNm = torqueSetpointNm;
telemetry.ready = ready;
[torquePayload, readyPayload] = packCarMakerTelemetry(telemetry);
end

== matlab function inverter_hil/Hardware I O - PRE-FLIGHT DISABLED/Pedal Fallback Zero Hold ==
  data: throttleIn input; throttleOut output; brakeIn input; canOwnsPedals input; brakeOut output
function [throttleOut,brakeOut] = pedalFallbackZeroHold( ...
    throttleIn, brakeIn, canOwnsPedals)
%PEDALFALLBACKZEROHOLD Hold the non-CAN pedal fallback at zero after
%CAN pedal authority is lost, until both GUI values return to zero.
%
%   Without this latch the source switches fall back to whatever the
%   GUI dictionary entries hold, so a slider left mid-travel would
%   step AO01-AO04 into the real VC the moment the CAN link dropped.
%   Zeroing in the GUI instead leaves a window one poll wide; this is
%   the model-side guarantee that closes it. Re-arming on the sliders
%   returning to zero keeps recovery automatic - no operator re-arm -
%   while making it impossible to resume at a stale non-zero demand.
%#codegen
persistent armed
if isempty(armed)
    armed = false;
end
zeroTolerance = 0.001;
if canOwnsPedals ~= 0
    % CAN is driving; the switches ignore these outputs. Arm so that the
    % next loss of authority is caught even if it happens next step.
    armed = true;
    throttleOut = throttleIn;
    brakeOut = brakeIn;
elseif armed
    if throttleIn <= zeroTolerance && brakeIn <= zeroTolerance
        armed = false;
        throttleOut = throttleIn;
        brakeOut = brakeIn;
    else
        throttleOut = 0;
        brakeOut = 0;
    end
else
    throttleOut = throttleIn;
    brakeOut = brakeIn;
end

== matlab function inverter_hil/Hardware I O - PRE-FLIGHT DISABLED/Pedal Voltage Calibration ==
  data: throttle input; ao1 output; brake input; released1 input; pressed1 input; released2 input; pressed2 input; released3 input; pressed3 input; released4 input; pressed4 input; ao2 output; ao3 output; ao4 output
function [ao1,ao2,ao3,ao4] = pedalVoltageCalibration( ...
    throttle, brake, released1, pressed1, released2, pressed2, ...
    released3, pressed3, released4, pressed4)
%PEDALVOLTAGECALIBRATION Map GUI throttle/brake fractions (0-1) to
%the four redundant IO183 analog-output voltages using the
%calibrated released/pressed endpoints.
%
%   HIL_CAL_PEDALS_RELEASED_V*/PRESSED_V* ship as NaN precisely so an
%   uncalibrated channel is detectable rather than silently plausible
%   (INVERTER_HIL_PLAN.MD S3.1 requires each endpoint be measured at
%   the connected VCU pin under load). An uncalibrated or out-of-range
%   channel therefore drives 0 V -- the same level the IO183 initial
%   and reset values use -- instead of propagating NaN into a DAC.
ao1 = calibratedVolts(released1, pressed1, throttle);
ao2 = calibratedVolts(released2, pressed2, throttle);
ao3 = calibratedVolts(released3, pressed3, brake);
ao4 = calibratedVolts(released4, pressed4, brake);
end

function volts = calibratedVolts(releasedV, pressedV, fraction)
if ~isfinite(releasedV) || ~isfinite(pressedV) || ~isfinite(fraction)
    volts = 0;
    return
end
bounded = min(max(fraction, 0), 1);
volts = releasedV + (pressedV - releasedV) * bounded;
%The IO183 analog outputs are configured for the 0..5 V range.
volts = min(max(volts, 0), 5);
end

== matlab function inverter_hil/Hardware I O - PRE-FLIGHT DISABLED/Precharge Pulse Generator ==
  data: counter input; active output
function active = prechargePulseFromCounter(counter)
%PRECHARGEPULSEFROMCOUNTER Turn a GUI counter increment into a
%fixed-width PRECH_BTN_IN pulse (INVERTER_HIL_PLAN.MD S7.1: "Model
%generates a deterministic precharge pulse on counter change").
%200 ms (at the model's 1 ms base rate) is provisional pending
%confirmation against VCU firmware precharge-button timing.
persistent prevCounter ticksRemaining initialized
pulseTicks = uint32(200);
if isempty(initialized)
    prevCounter = counter;
    ticksRemaining = uint32(0);
    initialized = true;
end
if counter ~= prevCounter
    ticksRemaining = pulseTicks;
    prevCounter = counter;
end
%Emitted as double because that is what the IO183 Digital Output
%port takes.
active = double(ticksRemaining > uint32(0));
if ticksRemaining > uint32(0)
    ticksRemaining = ticksRemaining - uint32(1);
end
end
